simulink model "model"  (R2013a)
settings: Solver=ode3  StartTime=0.0  StopTime=10.0  FixedStep=0.0001  MaxStep=0.2  MinStep=0.1  RelTol=1e-3
values from neighbouring files (symbols this model uses):
  d = 1    [skrypt.m]
  i = 1    [skrypt.m]
  tau = 0.01    [skrypt.m]
  x = 0    [skrypt.m]
undefined symbols (not defined in the file or in its folder): k, Td, Ti
settings Model: Creator=Dawid Perdek  LastModifiedBy=Dawid Perdek
settings SolverCC: InitialStep=0.2

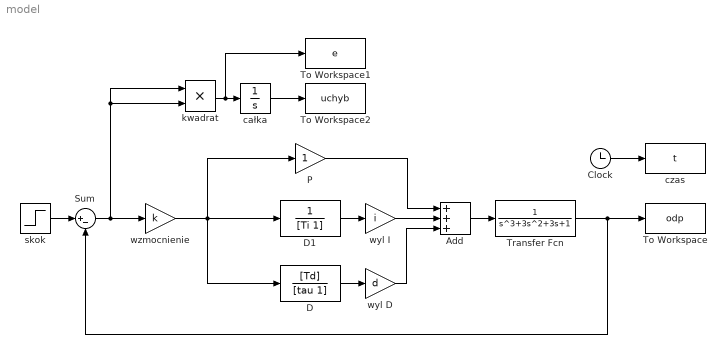
== system model ==
  Add : Sum  Inputs=+++
  Clock : Clock
  D : TransferFcn  Numerator=[Td]  Denominator=[tau 1]
  D1 : TransferFcn  Denominator=[Ti 1]
  P : Gain
  Sum : Sum  Inputs=|+-
  To Workspace : ToWorkspace  VariableName=odp  SampleTime=-1
  To Workspace1 : ToWorkspace  VariableName=e  SampleTime=-1
  To Workspace2 : ToWorkspace  VariableName=uchyb  SampleTime=-1
  Transfer Fcn : TransferFcn  Denominator=[1 3 3 1]
  całka : Integrator  UpperSaturationLimit=10  LowerSaturationLimit=0
  czas : ToWorkspace  VariableName=t  SampleTime=-1
  kwadrat : Product
  skok : Step  Time=x  SampleTime=0
  wyl D : Gain  Gain=d
  wyl I : Gain  Gain=i
  wzmocnienie : Gain  Gain=k
  wires:
  Transfer Fcn/1 -> Sum/2, To Workspace/1
  Add/1 -> Transfer Fcn/1
  P/1 -> Add/1
  skok/1 -> Sum/1
  Sum/1 -> wzmocnienie/1, kwadrat/2, kwadrat/1
  kwadrat/1 -> To Workspace1/1, całka/1
  całka/1 -> To Workspace2/1
  Clock/1 -> czas/1
  wzmocnienie/1 -> D1/1, D/1, P/1
  D1/1 -> wyl I/1
  D/1 -> wyl D/1
  wyl I/1 -> Add/2
  wyl D/1 -> Add/3
